simulink model "simulation_w_switch_sln3"  (Simulink 10.1)
settings: Solver=VariableStepAuto  StartTime=0.0  StopTime=tTot  MaxStep=1e-5  RelTol=1e-5
PreLoadFcn:
  | syst_init
values from neighbouring files (symbols this model uses):
  Aij = Aconn-Aii    [syst_init.m]
  AL = blkdiag(DGU.ALi)    [syst_init.m]
  atk24 = [zeros(3,1); 0.1*rand(3,1)-0.05]    [syst_init.m]
  atk34 = [zeros(3,1); 0.1*rand(3,1)-0.05]    [syst_init.m]
  B = blkdiag(DGU.B)    [syst_init.m]
  bC = blkdiag(DGU.bC)    [syst_init.m]
  bF = blkdiag(DGU.bF)    [syst_init.m]
  bH = blkdiag(DGU.bH)    [syst_init.m]
  bigCyComm = [zeros(3,3)  eye(3) zeros(3,30) ... (first row only)    [syst_init.m]
  bKhat = blkdiag(DGU.bKhat)    [syst_init.m]
  DGU = stateDyn(DGU,6)    [syst_init.m]
  F = blkdiag(DGU.Fj)    [syst_init.m]
  H = blkdiag(DGU.Hj)    [syst_init.m]
  K = blkdiag(DGU.K)    [syst_init.m]
  Khat = blkdiag(DGU.Khat)    [syst_init.m]
  L = blkdiag(DGU.Li)    [syst_init.m]
  n = 3    [syst_init.m]
  N = 6    [syst_init.m]
  nMaxMeas = .01    (= 0.01)    [syst_init.m]
  rhoMax = nMaxMeas*repmat([ones(n-1,1);0],N,1)    [syst_init.m]
  T = blkdiag(DGU.Tj)    [syst_init.m]
  Ta = 8    [syst_init.m]
  Tc = 2    [syst_init.m]
  tSampData = 1e-3    (= 0.001)    [syst_init.m]
  Vs = 60    [syst_init.m]
  wMax = nMax*repmat([ones(n-1,1);0],N,1)+nMaxMeas*repmat([zeros(n-1,1);1],N,1)    [syst_init.m]
undefined symbols (not defined in the file or in its folder): epsilon0bar, integral_Loc, rLoc_bar
libraries: powerlib x136, powerlib_meascontrol x13
(part 4 of 4)

== system simulation_w_switch_sln3/DGU6/UIO1 ==
  note: Single UIO for all neighbors of DGU 1 with Switched Inputs
  note: Calculated Switching Inputs
  note: 6x6 UIO for the states of DGUs with average dynamics
  Constant1 : Constant  Commented=on  Value=Vs
  Constant2 : Constant  Commented=on  Value=0.8132
  Divide : Product  Commented=on  Inputs=*/  Multiplication=Matrix(*)
  From5 : From  Commented=on  GotoTag=yComm6  TagVisibility=global
  From7 : From  Commented=on  GotoTag=yComm6  TagVisibility=global
  From8 : From  Commented=on  GotoTag=SW_yComm6  TagVisibility=global
  From9 : From  Commented=on  GotoTag=secondary  TagVisibility=global
  Gain15 : Gain  Gain=bH  Multiplication=Matrix(K*u) (u vector)
  Gain16 : Gain  Gain=inv(bC)-bH  Multiplication=Matrix(K*u) (u vector)
  Gain17 : Gain  Gain=bKhat  Multiplication=Matrix(K*u) (u vector)
  Gain18 : Gain  Gain=bF  Multiplication=Matrix(K*u) (u vector)
  Gain4 : Gain  Commented=on  Gain=K  Multiplication=Matrix(K*u) (u vector)
  Gain5 : Gain  Commented=on  Gain=[Khat T*B]  Multiplication=Matrix(K*u) (u vector)
  Gain6 : Gain  Commented=on  Gain=F  Multiplication=Matrix(K*u) (u vector)
  Gain7 : Gain  Commented=on  Gain=59.7999
  Gain8 : Gain  Commented=on  Gain=H  Multiplication=Matrix(K*u) (u vector)
  Gain9 : Gain  Commented=on  Gain=T  Multiplication=Matrix(K*u) (u vector)
  Goto : Goto  Commented=on  GotoTag=SW_yComm6  TagVisibility=global
  Goto3 : Goto  Commented=on  GotoTag=y_j6_hat  TagVisibility=global
  Goto4 : Goto  Commented=on  GotoTag=Duty_yComm6  TagVisibility=global
  Integrator1 : Integrator  Commented=on  ExternalReset=rising  InitialConditionSource=external
  Integrator4 : Integrator  ExternalReset=rising  InitialConditionSource=external  InitialCondition=[0;0;0]
  Mux3 : Mux  Commented=on  Inputs=2
  PWM Generator (DC-DC) : powerlib_meascontrol/Pulse & Signal Generators/PWM Generator (DC-DC)  Commented=on  Fsw=10000  Ts=0
  Product1 : Product  Commented=on  Multiplication=Matrix(*)
  Product4 : Product  Multiplication=Matrix(*)
  Sum10 : Sum  Inputs=++|
  Sum11 : Sum  Inputs=++|
  Sum2 : Sum  Commented=on  Inputs=++|
  Sum3 : Sum  Commented=on  Inputs=++|
  Sum4 : Sum  Commented=on  Inputs=|-+
  tag scope: xbar6=global
  wires:
  PWM Generator (DC-DC)/1 -> Goto/1
  Divide/1 -> Goto4/1, PWM Generator (DC-DC)/1
  Constant1/1 -> Divide/2
  Gain4/1 -> Divide/1
  From7/1 -> Gain4/1
  Constant2/1 -> Sum4/1
  From5/1 -> Gain8/1, Gain9/1, Mux3/1
  Sum3/1 -> Product1/1
  Gain5/1 -> Sum2/2
  Gain7/1 -> Sum4/2
  From8/1 -> Gain7/1
  Mux3/1 -> Gain5/1
  Gain8/1 -> Sum3/1
  Gain9/1 -> Integrator1/3
  From9/1 -> Integrator1/2, Product1/2
  Sum2/1 -> Integrator1/1
  Sum4/1 -> Mux3/2
  Integrator1/1 -> Sum3/2, Gain6/1
  Gain6/1 -> Sum2/1
  Product1/1 -> Goto3/1
  Sum11/1 -> Product4/1
  Gain17/1 -> Sum10/2
  Gain16/1 -> Integrator4/3
  Sum10/1 -> Integrator4/1
  [yComm6] -> Gain16/1, Gain15/1, Gain17/1
  Gain18/1 -> Sum10/1
  Gain15/1 -> Sum11/1
  Product4/1 -> [xbar6]
  Integrator4/1 -> Sum11/2, Gain18/1
  [secondary] -> Integrator4/2, Product4/2

== system simulation_w_switch_sln3/DGU1/Luenberger  Observer/Enabled  Luenberger ==
  u : Inport
  Enable : EnablePort  StatesWhenEnabling=reset
  xhat : Outport  VectorParamsAs1DForOutWhenUnconnected=off
  wires:
  ? -> xhat/1
  u/1 -> ?

== system simulation_w_switch_sln3/DGU1/UIO/Enabled  UIO ==
  u : Inport
  Enable : EnablePort  StatesWhenEnabling=reset
  State-Space : StateSpace  A=F  B=Khat  C=eye(n*N)  D=H  InitialCondition=zeros(n*N,1)
  y_ji_hat : Outport  VectorParamsAs1DForOutWhenUnconnected=off
  wires:
  u/1 -> State-Space/1
  State-Space/1 -> y_ji_hat/1

== matlab function Luenberger Thresholds/MATLAB Function ==
  data: u input double; y output double
function y = rLoc_bar(u)

gamma = (@(Tau) (abs(expm(AL*(u-Tc)))));
integrall = integral(gamma,Tc,u,'ArrayValued',true);
y = expm(AL*(u-Tc))*rhoMax + integrall*(abs(Aij)*rhoMax+wMax+abs(L)*rhoMax) + rhoMax;
